simulink model "bank_bootstrapping"  (R2020a)
settings: Solver=VariableStepAuto  StartTime=0.0  StopTime=10.0  RelTol=1e-3
values from neighbouring files (symbols this model uses):
  i_l = 0.075    [bank_and_economy.m]    (also in bank_centralbank.m = 0.055; bootstrapping.m = 0.055; main.m = 0.055)
  i_m = 0.03    [bank_and_economy.m]    (also in bank_centralbank.m; bootstrapping.m; main.m)
  K_0 = 0.08    [a_1.m]    (also in a_2.m; a_loss_function.m; bank_and_economy.m; bank_centralbank.m)
  K_p = 15    [a_1.m]    (also in a_2.m; a_loss_function.m; bank_and_economy.m = 0.5; bank_centralbank.m)
  lambda = 0.002    [a_1.m]    (also in a_2.m; a_loss_function.m; bank_and_economy.m; bank_centralbank.m)
  R = 1    [a_1.m]    (also in a_2.m; a_loss_function.m; bank_and_economy.m; bank_centralbank.m)
  rate = 0.1    [a_1.m]    (also in a_2.m; a_loss_function.m; bank_and_economy.m; bank_centralbank.m)
  sigma = 0.28    [a_1.m]    (also in a_2.m; a_loss_function.m; bank_and_economy.m; bank_centralbank.m)
  T_i = 8    [a_1.m]    (also in a_2.m; a_loss_function.m; bank_and_economy.m; bank_centralbank.m)
settings Model: Creator=erlended  LastModifiedBy=erlended

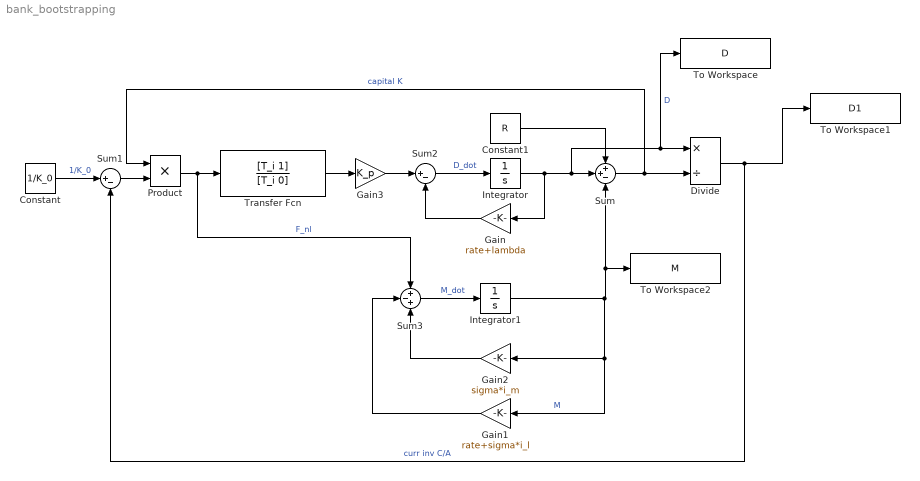
== system bank_bootstrapping ==
  Constant : Constant  Value=1/K_0
  Constant1 : Constant  Value=R
  Divide : Product  Inputs=*/
  Gain : Gain  Gain=rate+lambda
  Gain1 : Gain  Gain=rate+sigma*i_l
  Gain2 : Gain  Gain=sigma*i_m
  Gain3 : Gain  Gain=K_p
  Integrator : Integrator
  Integrator1 : Integrator
  Product : Product
  Sum : Sum  Inputs=++-
  Sum1 : Sum  Inputs=|+-
  Sum2 : Sum  Inputs=|+-
  Sum3 : Sum  Inputs=+-+
  To Workspace : ToWorkspace  VariableName=D  SaveFormat=Timeseries  SampleTime=-1
  To Workspace1 : ToWorkspace  VariableName=D1  SaveFormat=Timeseries  SampleTime=-1
  To Workspace2 : ToWorkspace  VariableName=M  SaveFormat=Timeseries  SampleTime=-1
  Transfer Fcn : TransferFcn  Numerator=[T_i 1]  Denominator=[T_i 0]
  wires:
  Product/1 -> Transfer Fcn/1, Sum3/1  "F_nl"
  Sum/1 -> Product/1, Divide/2  "capital K"
  Sum1/1 -> Product/2
  Constant/1 -> Sum1/1  "1/K_0"
  Transfer Fcn/1 -> Gain3/1
  Sum2/1 -> Integrator/1  "D_dot"
  Integrator/1 -> Gain/1, To Workspace/1, Divide/1, Sum/2  "D"
  Constant1/1 -> Sum/1
  Gain/1 -> Sum2/2
  Integrator1/1 -> Gain2/1, Gain1/1, To Workspace2/1, Sum/3  "M"
  Sum3/1 -> Integrator1/1  "M_dot"
  Gain1/1 -> Sum3/2
  Gain2/1 -> Sum3/3
  Divide/1 -> To Workspace1/1, Sum1/2  "curr inv C/A"
  Gain3/1 -> Sum2/1
